simulink model "HW5_e"  (R2024b)
settings: Solver=VariableStepAuto  StartTime=0.0  StopTime=50  RelTol=1e-3
values from neighbouring files (symbols this model uses):
  Kd = 0    [HW5.m]
  Ki = 3    [HW5.m]
  Kp = 0.5    [HW5.m]
  Ts = 0.001    [HW5.m]
libraries: slpidlib x1
settings Model: Creator=patrickstar  LastModifiedBy=patrickstar

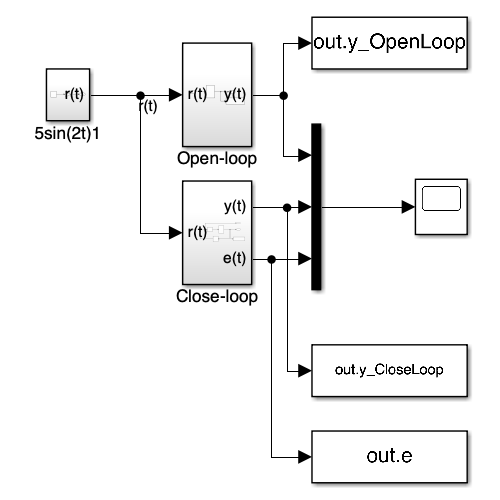
[thumbnail: Simulink's stored preview of the top-level diagram]
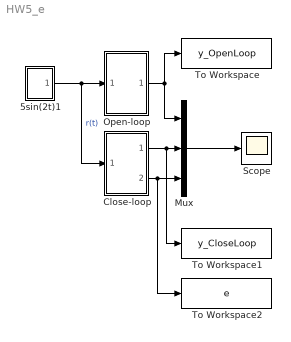
== system HW5_e ==
  5sin(2t)1 : Subsystem
  Close-loop : Subsystem
  Mux : Mux  Inputs=3
  Open-loop : Subsystem
  Scope : Scope
  To Workspace : ToWorkspace  VariableName=y_OpenLoop  SaveFormat=Timeseries  SampleTime=-1
  To Workspace1 : ToWorkspace  VariableName=y_CloseLoop  SaveFormat=Timeseries  SampleTime=-1
  To Workspace2 : ToWorkspace  VariableName=e  SaveFormat=Timeseries  SampleTime=-1
  wires:
  Close-loop/1(y(t)) -> To Workspace1/1, Mux/2
  Open-loop/1(y(t)) -> Mux/1, To Workspace/1
  Close-loop/2(e(t)) -> To Workspace2/1, Mux/3
  5sin(2t)1/1(r(t)) -> Open-loop/1(r(t)), Close-loop/1(r(t))  "r(t)"
  Mux/1 -> Scope/1

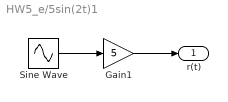
== system HW5_e/5sin(2t)1 ==
  Gain1 : Gain  Gain=5
  Sine Wave : Sin  Frequency=2  SampleTime=0
  r(t) : Outport
  wires:
  Gain1/1 -> r(t)/1
  Sine Wave/1 -> Gain1/1

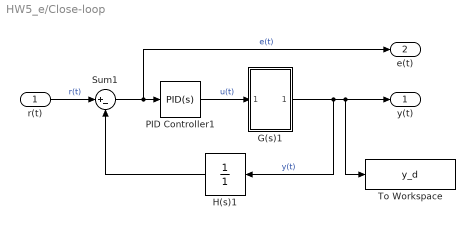
== system HW5_e/Close-loop ==
  r(t) : Inport
  G(s)1 : Subsystem
  H(s)1 : TransferFcn  Denominator=[1]
  PID Controller1 : slpidlib/PID Controller  Controller=PID  Form=Parallel  TimeDomain=Continuous-time  UseExternalTs=off  SampleTime=-1  IntegratorMethod=Forward Euler  FilterMethod=Forward Euler  ControllerParametersSource=internal  P=Kp  I=Ki  UseKiTs=off  D=Kd  UseExternalDerivativeSource=off  N=100  UseFilter=on  TunerSelectOption=Transfer Function Based (PID Tuner App)  InitialConditionSource=internal  InitialConditionForIntegrator=0  InitialConditionForFilter=0  DifferentiatorICPrevScaledInput=0  ExternalReset=none  TrackingMode=off  Kt=1  LimitOutput=off  SatLimitsSource=internal  UpperSaturationLimit=inf  LowerSaturationLimit=-inf  LinearizeAsGain=on  AntiWindupMode=none  Kb=1  LimitIntegrator=off  UpperIntegratorSaturationLimit=inf  LowerIntegratorSaturationLimit=-inf  POutMin=[]  POutMax=[]  IOutMin=[]  IOutMax=[]  DOutMin=[]  DOutMax=[]  NOutMin=[]  NOutMax=[]  SumOutMin=[]  SumOutMax=[]  SaturationOutMin=[]  SaturationOutMax=[]  PParamMin=[]  PParamMax=[]  IParamMin=[]  IParamMax=[]  DParamMin=[]  DParamMax=[]  NParamMin=[]  NParamMax=[]  KbParamMin=[]  KbParamMax=[]  KtParamMin=[]  KtParamMax=[]  KbOutMin=[]  KbOutMax=[]  KtOutMin=[]  KtOutMax=[]  IntegratorOutMin=[]  IntegratorOutMax=[]  FilterOutMin=[]  FilterOutMax=[]  SumI1OutMin=[]  SumI1OutMax=[]  SumI2OutMin=[]  SumI2OutMax=[]  SumI3OutMin=[]  SumI3OutMax=[]  SumI4OutMin=[]  SumI4OutMax=[]  SumDOutMin=[]  SumDOutMax=[]  DifferentiatorOutMin=[]  DifferentiatorOutMax=[]  FilterDiffOutCoefMin=[]  FilterDiffOutCoefMax=[]  ReciprocalOutMin=[]  ReciprocalOutMax=[]  SumDenOutMin=[]  SumDenOutMax=[]  SumNumOutMin=[]  SumNumOutMax=[]  DivideOutMin=[]  DivideOutMax=[]  UdiffTsProdOutMin=[]  UdiffTsProdOutMax=[]  NTsProdOutMin=[]  NTsProdOutMax=[]  UintegralTsProdOutMin=[]  UintegralTsProdOutMax=[]  UngainTsProdOutMin=[]  UngainTsProdOutMax=[]  ClampingZeroOutDataTypeStr=Inherit: Inherit via back propagation  ClampingZeroOutMin=[]  ClampingZeroOutMax=[]  FilterDenConstantOutDataTypeStr=Inherit: Inherit via back propagation  FilterDenConstantOutMin=[]  FilterDenConstantOutMax=[]  PCopyOutDataTypeStr=Inherit: Inherit via back propagation  PCopyOutMin=[]  PCopyOutMax=[]  NCopyOutDataTypeStr=Inherit: Inherit via back propagation  NCopyOutMin=[]  NCopyOutMax=[]  IntegratorContinuousStateAttributes=''  IntegratorStateMustResolveToSignalObject=off  IntegratorRTWStateStorageClass=Auto  FilterContinuousStateAttributes=''  FilterStateMustResolveToSignalObject=off  FilterRTWStateStorageClass=Auto  ParallelPVariant=InternalParameters  IdealPVariant=Disabled  IVariant=InternalParameters  DVariant=InternalParameters  IntegratorVariant=Continuous  SatVariant=Disabled  AWVariant=Passthrough  PCopyVariant=Disabled  TRVariant=Disabled  FdbkBlocksVariant=Forward  IdealPFdbkVariant=Disabled  SatFdbkVariant=Disabled  DerivativeFilterVariant=ContFilter  NVariant=InternalParameters  NCopyVariant=Disabled  FilterICVariant=InternalICsFilter  IntegratorICVariant=InternalICs  ExternalResetVariant=Disabled  TRSumVariant=Passthrough  SumFdbkVariant=Disabled  SumVariant=Sum_PID  TsampFilterVariant=InternalTs  TsampNgainVariant=Passthrough  TsampIntegralVariant=Disabled_SignalSpec  ExternalSaturationOutDataTypeStr=Inherit: Same as second input  DerivativeSourceVariant=ErrorSignal  PreIntVariant=InternalPreInt
  Sum1 : Sum  Inputs=|+-
  To Workspace : ToWorkspace  VariableName=y_d  SaveFormat=Timeseries  SampleTime=Ts
  y(t) : Outport
  e(t) : Outport  Port=2
  wires:
  H(s)1/1 -> Sum1/2
  r(t)/1 -> Sum1/1  "r(t)"
  Sum1/1 -> e(t)/1, PID Controller1/1  "e(t)"
  PID Controller1/1 -> G(s)1/1(u(t))  "u(t)"
  G(s)1/1(y(t)) -> y(t)/1, To Workspace/1, H(s)1/1  "y(t)"

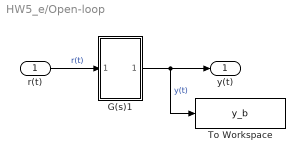
== system HW5_e/Open-loop ==
  r(t) : Inport
  G(s)1 : Subsystem
  To Workspace : ToWorkspace  VariableName=y_b  SaveFormat=Timeseries  SampleTime=-1
  y(t) : Outport
  wires:
  G(s)1/1(y(t)) -> y(t)/1, To Workspace/1  "y(t)"
  r(t)/1 -> G(s)1/1(r(t))  "r(t)"

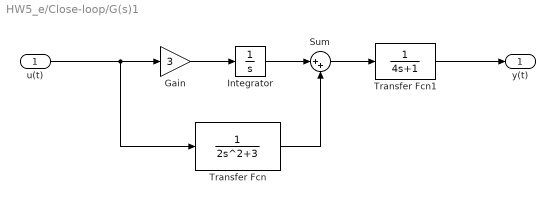
== system HW5_e/Close-loop/G(s)1 ==
  u(t) : Inport
  Gain : Gain  Gain=3
  Integrator : Integrator
  Sum : Sum  Inputs=|++
  Transfer Fcn : TransferFcn  Denominator=[2 0 3]
  Transfer Fcn1 : TransferFcn  Denominator=[4 1]
  y(t) : Outport
  wires:
  Transfer Fcn/1 -> Sum/2
  u(t)/1 -> Transfer Fcn/1, Gain/1
  Sum/1 -> Transfer Fcn1/1
  Integrator/1 -> Sum/1
  Transfer Fcn1/1 -> y(t)/1
  Gain/1 -> Integrator/1

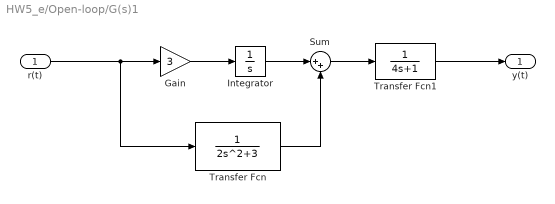
== system HW5_e/Open-loop/G(s)1 ==
  r(t) : Inport
  Gain : Gain  Gain=3
  Integrator : Integrator
  Sum : Sum  Inputs=|++
  Transfer Fcn : TransferFcn  Denominator=[2 0 3]
  Transfer Fcn1 : TransferFcn  Denominator=[4 1]
  y(t) : Outport
  wires:
  Transfer Fcn/1 -> Sum/2
  r(t)/1 -> Transfer Fcn/1, Gain/1
  Sum/1 -> Transfer Fcn1/1
  Integrator/1 -> Sum/1
  Transfer Fcn1/1 -> y(t)/1
  Gain/1 -> Integrator/1
